simulink model "task9_lab12"  (R2021a)
settings: Solver=VariableStepAuto  StartTime=0.0  StopTime=10.0  RelTol=1e-3
undefined symbols (not defined in the file): Call, Function
settings Model: Creator=reemb  LastModifiedBy=reemb

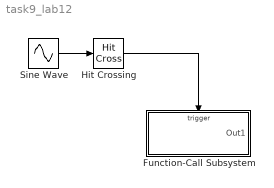
== system task9_lab12 ==
  Function-Call Subsystem : Subsystem  TreatAsAtomicUnit=on
  Hit Crossing : HitCross  HitCrossingDirection=falling  HitCrossingOutputType=Function-Call
  Sine Wave : Sin  SampleTime=0
  wires:
  Sine Wave/1 -> Hit Crossing/1
  Hit Crossing/1 -> Function-Call Subsystem/Trigger

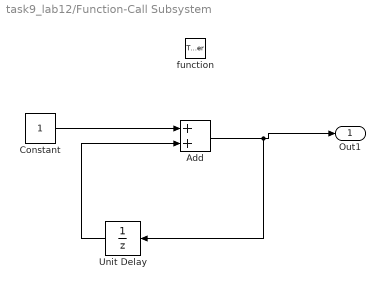
== system task9_lab12/Function-Call Subsystem ==
  function : TriggerPort  TriggerType=function-call  VariantControl=(inherit)
  Add : Sum
  Constant : Constant
  Unit Delay : UnitDelay  SampleTime=-1  HasFrameUpgradeWarning=on
  Out1 : Outport
  wires:
  Constant/1 -> Add/1
  Add/1 -> Unit Delay/1, Out1/1
  Unit Delay/1 -> Add/2
